simulink model "dynsim_2link_planar"  (R2020a)
settings: Solver=ode3  StartTime=0.0  StopTime=10.0  FixedStep=0.05  RelTol=1e-3
undefined symbols (not defined in the file or in its folder): Header, Pose, Twist
libraries: robotlib x21, robotmaniplib x3
settings Model: Creator=ROS_PO  LastModifiedBy=paolo
settings OptimizationCC: EnhancedBackFolding=on  PassReuseOutputArgsAs=Individual arguments  ZeroExternalMemoryAtStartup=off  ZeroInternalMemoryAtStartup=off  MaxStackSize=64  OptimizeBlockOrder=speed  DifferentSizesBufferReuse=on  OptimizationCustomize=off  EfficientTunableParamExpr=on
settings DebuggingCC: ParameterTunabilityLossMsg=error
settings HardwareCC: ProdBitPerPointer=32  ProdBitPerSizeT=32  ProdBitPerPtrDiffT=32  ProdLargestAtomicFloat=None  ProdIntDivRoundTo=Undefined  ProdEndianess=Unspecified  ProdWordSize=32  ProdHWDeviceType=Generic->Unspecified (assume 32-bit Generic)
settings RTWCC: SystemTargetFile=ert.tlc  HardwareBoard=Robot Operating System (ROS)  TemplateMakefile=ert_default_tmf  GenerateReport=on  Toolchain=Catkin  IncludeHyperlinkInReport=on  LaunchReport=on  TargetLang=C++  GenerateTraceInfo=on  GenerateTraceReport=on  GenerateTraceReportSl=on  GenerateTraceReportSf=on  GenerateTraceReportEml=on
settings CodeAppCC: ForceParamTrailComments=on  IgnoreCustomStorageClasses=off  OperatorAnnotations=on  SimulinkDataObjDesc=on  SFDataObjDesc=on  InsertBlockDesc=on
settings ERTTargetCC: SupportContinuousTime=on  SupportVariableSizeSignals=on

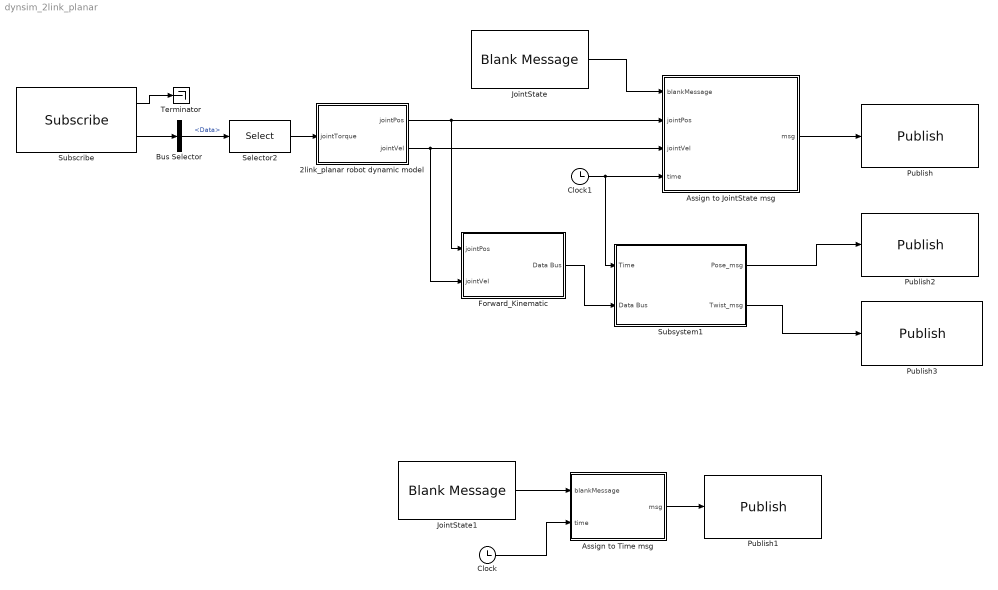
== system dynsim_2link_planar ==
  2link_planar robot dynamic model : Subsystem
  Assign to JointState msg : MATLAB Function  TreatAsAtomicUnit=on
  Assign to Time msg : MATLAB Function  TreatAsAtomicUnit=on
  Bus Selector : BusSelector  OutputSignals=Data
  Clock : Clock
  Clock1 : Clock
  Forward_Kinematic : Subsystem
  JointState : robotlib/Blank Message  messageClass=Message  entityType=sensor_msgs/JointState  messageType=sensor_msgs/JointState  SampleTime=inf
  JointState1 : robotlib/Blank Message  messageClass=Message  entityType=rosgraph_msgs/Clock  messageType=rosgraph_msgs/Clock  SampleTime=inf
  Publish : robotlib/Publish  topicSource=Specify your own  topic=/joint_states  messageType=sensor_msgs/JointState  messageQueueLength=1
  Publish1 : robotlib/Publish  topicSource=Specify your own  topic=/clock  messageType=rosgraph_msgs/Clock  messageQueueLength=1
  Publish2 : robotlib/Publish  topicSource=Specify your own  topic=/cartesian_pos  messageType=geometry_msgs/PoseStamped  messageQueueLength=1
  Publish3 : robotlib/Publish  topicSource=Specify your own  topic=/cartesian_vel  messageType=geometry_msgs/TwistStamped  messageQueueLength=1
  Selector2 : Selector  IndexOptions=Starting index (dialog)  Indices=[2]  OutputSizes=6
  Subscribe : robotlib/Subscribe  topicSource=Specify your own  topic=/joint_torque  messageType=std_msgs/Float64MultiArray  sampleTime=-1  messageQueueLength=1
  Subsystem1 : Subsystem
  Terminator : Terminator
  wires:
  2link_planar robot dynamic model/2(jointVel) -> Forward_Kinematic/2(jointVel), Assign to JointState msg/3(jointVel)
  Assign to JointState msg/1(msg) -> Publish/1
  Clock1/1 -> Subsystem1/1(Time), Assign to JointState msg/4(time)
  JointState1/1 -> Assign to Time msg/1(blankMessage)
  Selector2/1 -> 2link_planar robot dynamic model/1(jointTorque)
  Subscribe/1 -> Terminator/1
  Subscribe/2 -> Bus Selector/1
  2link_planar robot dynamic model/1(jointPos) -> Assign to JointState msg/2(jointPos), Forward_Kinematic/1(jointPos)
  Bus Selector/1 -> Selector2/1  "<Data>"
  Clock/1 -> Assign to Time msg/2(time)
  Assign to Time msg/1(msg) -> Publish1/1
  JointState/1 -> Assign to JointState msg/1(blankMessage)
  Subsystem1/2(Twist_msg) -> Publish3/1
  Forward_Kinematic/1(Data Bus) -> Subsystem1/2(Data Bus)
  Subsystem1/1(Pose_msg) -> Publish2/1

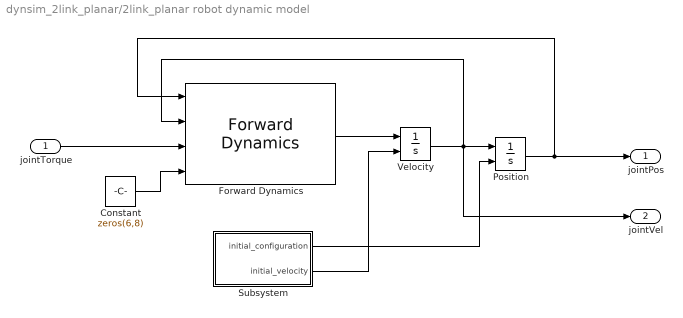
== system dynsim_2link_planar/2link_planar robot dynamic model ==
  jointTorque : Inport
  Constant : Constant  Value=zeros(6,8)
  Forward Dynamics : robotmaniplib/Forward Dynamics  RigidBodyTree=robot_2link_planar  SimulateUsing=Interpreted execution
  Position : Integrator  InitialConditionSource=external
  Subsystem : Subsystem
  Velocity : Integrator  InitialConditionSource=external
  jointPos : Outport
  jointVel : Outport  Port=2
  wires:
  Forward Dynamics/1 -> Velocity/1
  Position/1 -> Forward Dynamics/1, jointPos/1
  jointTorque/1 -> Forward Dynamics/3
  Constant/1 -> Forward Dynamics/4
  Velocity/1 -> Forward Dynamics/2, Position/1, jointVel/1
  Subsystem/2(initial_velocity) -> Velocity/2
  Subsystem/1(initial_configuration) -> Position/2

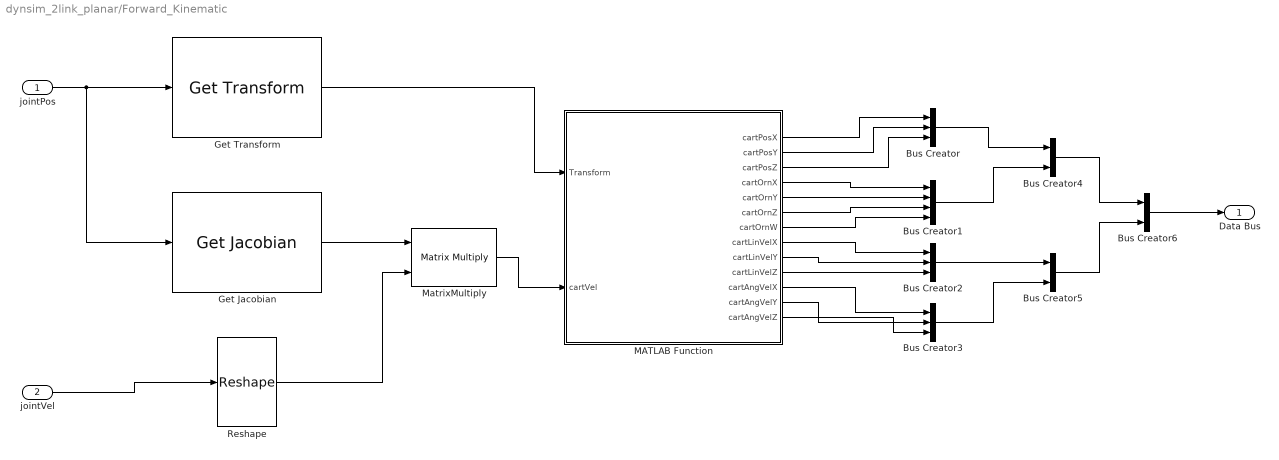
== system dynsim_2link_planar/Forward_Kinematic ==
  jointPos : Inport
  jointVel : Inport  Port=2
  Bus Creator : BusCreator  Inputs=3
  Bus Creator1 : BusCreator  Inputs=4
  Bus Creator2 : BusCreator  Inputs=3
  Bus Creator3 : BusCreator  Inputs=3
  Bus Creator4 : BusCreator  Inputs=2
  Bus Creator5 : BusCreator  Inputs=2
  Bus Creator6 : BusCreator  Inputs=2
  Get Jacobian : robotmaniplib/Get Jacobian  RigidBodyTree=robot_2link_planar  EndEffector=edo_link_ee  SimulateUsing=Interpreted execution
      settings: SourceProductBaseCode=RO
  Get Transform : robotmaniplib/Get Transform  RigidBodyTree=robot_2link_planar  SourceBody=world  TargetBody=edo_link_ee  SimulateUsing=Interpreted execution
  MATLAB Function : MATLAB Function  TreatAsAtomicUnit=on
  MatrixMultiply : Product  Multiplication=Matrix(*)
  Reshape : Reshape  OutputDimensionality=Column vector (2-D)
  Data Bus : Outport
  wires:
  jointPos/1 -> Get Jacobian/1, Get Transform/1
  Get Jacobian/1 -> MatrixMultiply/1
  jointVel/1 -> Reshape/1
  Reshape/1 -> MatrixMultiply/2
  MatrixMultiply/1 -> MATLAB Function/2(cartVel)
  Get Transform/1 -> MATLAB Function/1(Transform)
  MATLAB Function/1(cartPosX) -> Bus Creator/1
  MATLAB Function/2(cartPosY) -> Bus Creator/2
  MATLAB Function/3(cartPosZ) -> Bus Creator/3
  MATLAB Function/4(cartOrnX) -> Bus Creator1/1
  MATLAB Function/5(cartOrnY) -> Bus Creator1/2
  MATLAB Function/6(cartOrnZ) -> Bus Creator1/3
  MATLAB Function/7(cartOrnW) -> Bus Creator1/4
  MATLAB Function/8(cartLinVelX) -> Bus Creator2/1
  MATLAB Function/9(cartLinVelY) -> Bus Creator2/2
  MATLAB Function/10(cartLinVelZ) -> Bus Creator2/3
  MATLAB Function/11(cartAngVelX) -> Bus Creator3/1
  MATLAB Function/12(cartAngVelY) -> Bus Creator3/2
  MATLAB Function/13(cartAngVelZ) -> Bus Creator3/3
  Bus Creator/1 -> Bus Creator4/1
  Bus Creator1/1 -> Bus Creator4/2
  Bus Creator2/1 -> Bus Creator5/1
  Bus Creator3/1 -> Bus Creator5/2
  Bus Creator4/1 -> Bus Creator6/1
  Bus Creator5/1 -> Bus Creator6/2
  Bus Creator6/1 -> Data Bus/1

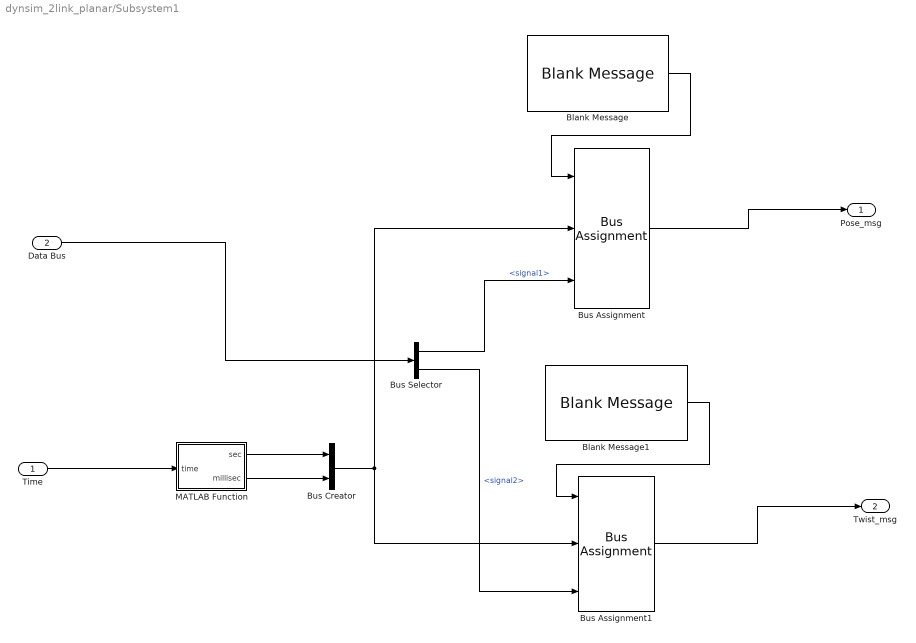
== system dynsim_2link_planar/Subsystem1 ==
  Time : Inport
  Data Bus : Inport  Port=2
  Blank Message : robotlib/Blank Message  messageClass=Message  entityType=geometry_msgs/PoseStamped  messageType=geometry_msgs/PoseStamped  SampleTime=inf
  Blank Message1 : robotlib/Blank Message  messageClass=Message  entityType=geometry_msgs/TwistStamped  messageType=geometry_msgs/TwistStamped  SampleTime=inf
  Bus Assignment : BusAssignment  AssignedSignals=Header.Stamp,Pose
  Bus Assignment1 : BusAssignment  AssignedSignals=Header.Stamp,Twist
  Bus Creator : BusCreator  Inputs=2
  Bus Selector : BusSelector  OutputSignals=signal1,signal2
  MATLAB Function : MATLAB Function  TreatAsAtomicUnit=on
  Pose_msg : Outport
  Twist_msg : Outport  Port=2
  wires:
  Blank Message/1 -> Bus Assignment/1
  Blank Message1/1 -> Bus Assignment1/1
  Data Bus/1 -> Bus Selector/1
  Bus Selector/1 -> Bus Assignment/3  "<signal1>"
  Bus Selector/2 -> Bus Assignment1/3  "<signal2>"
  MATLAB Function/1(sec) -> Bus Creator/1
  MATLAB Function/2(millisec) -> Bus Creator/2
  Bus Creator/1 -> Bus Assignment/2, Bus Assignment1/2
  Bus Assignment/1 -> Pose_msg/1
  Bus Assignment1/1 -> Twist_msg/1
  Time/1 -> MATLAB Function/1(time)

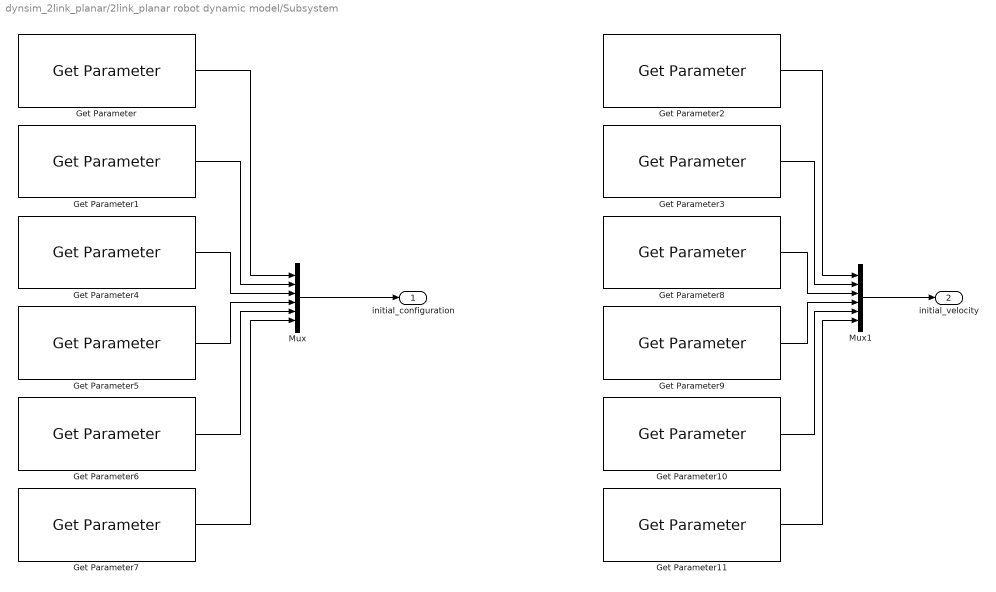
== system dynsim_2link_planar/2link_planar robot dynamic model/Subsystem ==
  Get Parameter : robotlib/Get Parameter  ParameterSource=Specify your own  ParameterName=/q1_initial  ParameterType=double  ParameterMaxArrayLength=16  ParameterInitialValue=0  SampleTime=-1  ShowErrorCodeOutput=off  ModelName=dynsim_2link_planar  BlockId=ParamGet_dynsim_2link_planar_131
      settings: SourceProductBaseCode=RR
  Get Parameter1 : robotlib/Get Parameter  ParameterSource=Specify your own  ParameterName=/q2_initial  ParameterType=double  ParameterMaxArrayLength=16  ParameterInitialValue=0  SampleTime=-1  ShowErrorCodeOutput=off  ModelName=dynsim_2link_planar  BlockId=ParamGet_dynsim_2link_planar_132
      settings: SourceProductBaseCode=RR
  Get Parameter10 : robotlib/Get Parameter  ParameterSource=Specify your own  ParameterName=/qv5_initial  ParameterType=double  ParameterMaxArrayLength=16  ParameterInitialValue=0  SampleTime=-1  ShowErrorCodeOutput=off  ModelName=dynsim_2link_planar  BlockId=ParamGet_dynsim_2link_planar_133
      settings: SourceProductBaseCode=RR
  Get Parameter11 : robotlib/Get Parameter  ParameterSource=Specify your own  ParameterName=/qv6_initial  ParameterType=double  ParameterMaxArrayLength=16  ParameterInitialValue=0  SampleTime=-1  ShowErrorCodeOutput=off  ModelName=dynsim_2link_planar  BlockId=ParamGet_dynsim_2link_planar_134
      settings: SourceProductBaseCode=RR
  Get Parameter2 : robotlib/Get Parameter  ParameterSource=Specify your own  ParameterName=/qv1_initial  ParameterType=double  ParameterMaxArrayLength=16  ParameterInitialValue=0  SampleTime=-1  ShowErrorCodeOutput=off  ModelName=dynsim_2link_planar  BlockId=ParamGet_dynsim_2link_planar_135
      settings: SourceProductBaseCode=RR
  Get Parameter3 : robotlib/Get Parameter  ParameterSource=Specify your own  ParameterName=/qv2_initial  ParameterType=double  ParameterMaxArrayLength=16  ParameterInitialValue=0  SampleTime=-1  ShowErrorCodeOutput=off  ModelName=dynsim_2link_planar  BlockId=ParamGet_dynsim_2link_planar_136
      settings: SourceProductBaseCode=RR
  Get Parameter4 : robotlib/Get Parameter  ParameterSource=Specify your own  ParameterName=/q3_initial  ParameterType=double  ParameterMaxArrayLength=16  ParameterInitialValue=0  SampleTime=-1  ShowErrorCodeOutput=off  ModelName=dynsim_2link_planar  BlockId=ParamGet_dynsim_2link_planar_137
      settings: SourceProductBaseCode=RR
  Get Parameter5 : robotlib/Get Parameter  ParameterSource=Specify your own  ParameterName=/q4_initial  ParameterType=double  ParameterMaxArrayLength=16  ParameterInitialValue=0  SampleTime=-1  ShowErrorCodeOutput=off  ModelName=dynsim_2link_planar  BlockId=ParamGet_dynsim_2link_planar_138
      settings: SourceProductBaseCode=RR
  Get Parameter6 : robotlib/Get Parameter  ParameterSource=Specify your own  ParameterName=/q5_initial  ParameterType=double  ParameterMaxArrayLength=16  ParameterInitialValue=0  SampleTime=-1  ShowErrorCodeOutput=off  ModelName=dynsim_2link_planar  BlockId=ParamGet_dynsim_2link_planar_139
      settings: SourceProductBaseCode=RR
  Get Parameter7 : robotlib/Get Parameter  ParameterSource=Specify your own  ParameterName=/q6_initial  ParameterType=double  ParameterMaxArrayLength=16  ParameterInitialValue=0  SampleTime=-1  ShowErrorCodeOutput=off  ModelName=dynsim_2link_planar  BlockId=ParamGet_dynsim_2link_planar_140
      settings: SourceProductBaseCode=RR
  Get Parameter8 : robotlib/Get Parameter  ParameterSource=Specify your own  ParameterName=/qv3_initial  ParameterType=double  ParameterMaxArrayLength=16  ParameterInitialValue=0  SampleTime=-1  ShowErrorCodeOutput=off  ModelName=dynsim_2link_planar  BlockId=ParamGet_dynsim_2link_planar_141
      settings: SourceProductBaseCode=RR
  Get Parameter9 : robotlib/Get Parameter  ParameterSource=Specify your own  ParameterName=/qv4_initial  ParameterType=double  ParameterMaxArrayLength=16  ParameterInitialValue=0  SampleTime=-1  ShowErrorCodeOutput=off  ModelName=dynsim_2link_planar  BlockId=ParamGet_dynsim_2link_planar_142
      settings: SourceProductBaseCode=RR
  Mux : Mux  Inputs=6
  Mux1 : Mux  Inputs=6
  initial_configuration : Outport
  initial_velocity : Outport  Port=2
  wires:
  Mux/1 -> initial_configuration/1
  Get Parameter/1 -> Mux/1
  Get Parameter1/1 -> Mux/2
  Get Parameter3/1 -> Mux1/2
  Get Parameter2/1 -> Mux1/1
  Mux1/1 -> initial_velocity/1
  Get Parameter4/1 -> Mux/3
  Get Parameter5/1 -> Mux/4
  Get Parameter6/1 -> Mux/5
  Get Parameter7/1 -> Mux/6
  Get Parameter8/1 -> Mux1/3
  Get Parameter9/1 -> Mux1/4
  Get Parameter10/1 -> Mux1/5
  Get Parameter11/1 -> Mux1/6

== matlab function dynsim_2link_planar/Assign to Time msg ==
  data: blankMessage input; msg output Bus: SL_Bus_dynsim_2link_planar_rosgraph_msgs_Clock; time input
function msg = assign_Time(blankMessage,time)
%#codegen

% Assign the output message to be the same with input blank message
msg = blankMessage;

% Convert and set time
msg.Clock_.Sec  = fix(time);
msg.Clock_.Nsec = fix((time-fix(time))*1e9);

== matlab function dynsim_2link_planar/Assign to JointState msg ==
  data: blankMessage input; msg output Bus: SL_Bus_dynsim_2link_planar_sensor_msgs_JointState; jointPos input; jointVel input; time input
function msg = assign_JointState(blankMessage,jointPos,jointVel,time)
%#codegen

% Assign the output message to be the same with input blank message
msg = blankMessage;

% Initialize time stamp
msg.Header.Stamp.Sec  = fix(time);
msg.Header.Stamp.Nsec = fix((time-fix(time))*1e9);

% Set the number of strings in the string array, and joint positions/velocities in the position/velocity array
numJoints = length(jointPos);
msg.Name_SL_Info.CurrentLength = uint32(numJoints);
msg.Position_SL_Info.CurrentLength = uint32(numJoints);
msg.Velocity_SL_Info.CurrentLength = uint32(numJoints);

% Set the individual components in the message arrays
strArrayToAssign = {'edo_joint_1', 'edo_joint_2', 'edo_joint_3', 'edo_joint_4', 'edo_joint_5', 'edo_joint_6'};

for idx=1:numJoints
    str = strArrayToAssign{idx};
    strLength = length(str);
    msg.Name(idx).Data(1:strLength) = uint8(str);
    msg.Name(idx).Data_SL_Info.CurrentLength = uint32(strLength);

    msg.Position(idx) = jointPos(idx);
    msg.Velocity(idx) = jointVel(idx);
end

== matlab function dynsim_2link_planar/Subsystem1/MATLAB Function ==
  data: time input; sec output; millisec output
function [sec, millisec] = fcn(time)

    sec = fix(time);
    millisec = fix((time - fix(time)) * 1e9);

== matlab function dynsim_2link_planar/Forward_Kinematic/MATLAB Function ==
  data: Transform input; cartPosX output; cartVel input; cartPosY output; cartPosZ output; cartOrnX output; cartOrnY output; cartOrnZ output; cartOrnW output; cartLinVelX output; cartLinVelY output; cartLinVelZ output; cartAngVelX output; cartAngVelY output; cartAngVelZ output
function [cartPosX, cartPosY, cartPosZ, cartOrnX, cartOrnY, cartOrnZ, cartOrnW, cartLinVelX, cartLinVelY, cartLinVelZ, cartAngVelX, cartAngVelY, cartAngVelZ] = calculate_cartesian_state(Transform, cartVel)

    cartPos = Transform(1:3, 4);
    temp = rotm2eul(Transform(1:3, 1:3));
    cartOrn = rotm2quat(Transform(1:3, 1:3));

    R = [0, -sin(temp(1)), cos(temp(1))*sin(temp(2)); %Matrix needed to go from geometric Jacobian to analytic Jacobian
         0, cos(temp(1)), sin(temp(1))*sin(temp(2)); 
         1, 0, cos(temp(2))];
 
    cartLinVel = cartVel(4:6);
    cartAngVel = cartVel(1:3);
    
    cartPosX = cartPos(1);
    cartPosY = cartPos(2);
    cartPosZ = cartPos(3);
    
    cartOrnX = cartOrn(1);
    cartOrnY = cartOrn(2);
    cartOrnZ = cartOrn(3);
    cartOrnW = cartOrn(4);
    
    cartLinVelX = cartLinVel(1);
    cartLinVelY = cartLinVel(2);
    cartLinVelZ = cartLinVel(3);
    
    cartAngVelX = cartAngVel(1);
    cartAngVelY = cartAngVel(2);
    cartAngVelZ = cartAngVel(3);
